simulink subsystem "bh_COMPONENT_deriv_est"  (R2022b)
settings: Solver=VariableStepAuto  StartTime=0.0  StopTime=10.0  RelTol=1e-3
model mask{wn=0, p=0}
  mask prompts: wn "Natural frequency, wn (rad/sec)"; p "Damping Ratio, p"
settings Model: Creator=bhorton  LastModifiedBy=bhorton
settings DebuggingCC: UnconnectedInputMsg=warning  UnconnectedOutputMsg=warning  UnconnectedLineMsg=warning
settings ModelReferenceCC: EnableRefExpFcnMdlSchedulingChecks=on
settings RTWCC: DLArmComputeVersion=19.05

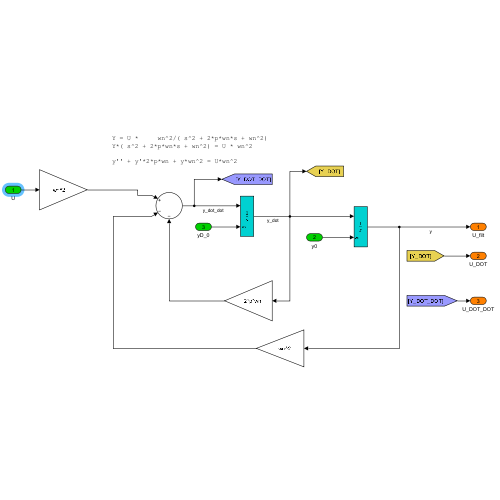
[thumbnail: Simulink's stored preview of the top-level diagram]
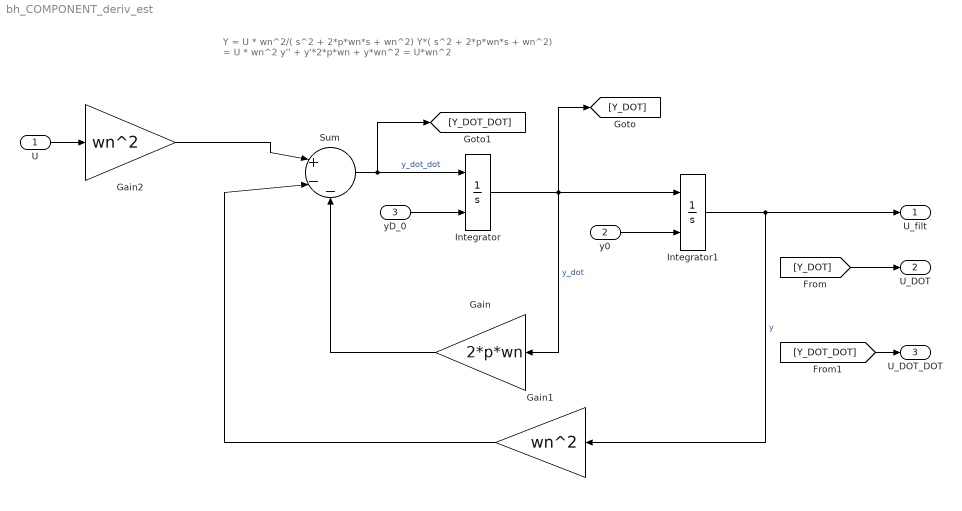
== system bh_COMPONENT_deriv_est ==
  note: Y = U *     wn^2/( s^2 + 2*p*wn*s + wn^2)
      | Y*( s^2 + 2*p*wn*s + wn^2) = U * wn^2
      |
      | y'' + y'*2*p*wn + y*wn^2 = U*wn^2
  U : Inport
  y0 : Inport  Port=2
  yD_0 : Inport  Port=3
  Gain : Gain  Gain=2*p*wn
  Gain1 : Gain  Gain=wn^2
  Gain2 : Gain  Gain=wn^2
  Integrator : Integrator  InitialConditionSource=external
  Integrator1 : Integrator  InitialConditionSource=external
  Sum : Sum  Inputs=|+--
  U_filt : Outport  VectorParamsAs1DForOutWhenUnconnected=off
  U_DOT : Outport  Port=2  VectorParamsAs1DForOutWhenUnconnected=off
  U_DOT_DOT : Outport  Port=3  VectorParamsAs1DForOutWhenUnconnected=off
  wires:
  y0/1 -> Integrator1/2
  yD_0/1 -> Integrator/2
  Sum/1 -> Integrator/1, [Y_DOT_DOT]  "y_dot_dot"
  Integrator/1 -> [Y_DOT], Gain/1, Integrator1/1  "y_dot"
  U/1 -> Gain2/1
  Gain1/1 -> Sum/2
  [Y_DOT] -> U_DOT/1
  Gain2/1 -> Sum/1
  Gain/1 -> Sum/3
  Integrator1/1 -> Gain1/1, U_filt/1  "y"
  [Y_DOT_DOT] -> U_DOT_DOT/1
